simulink model "simdecod5g1"  (R2023b)
settings: Solver=VariableStepAuto  StartTime=0.0  StopTime=0.01  RelTol=1e-3
undefined symbols (not defined in the file): waveform
libraries: commdigbbndam3 x3, commofdm x3
settings Model: Creator=joshua  LastModifiedBy=joshua

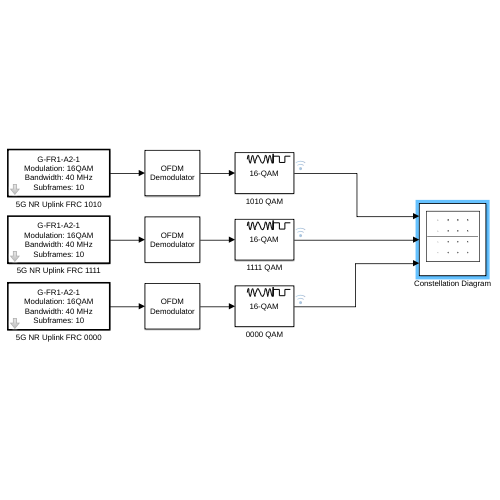
[thumbnail: Simulink's stored preview of the top-level diagram]
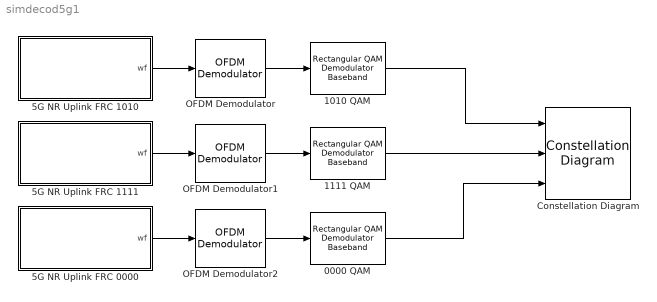
== system simdecod5g1 ==
  "0000 QAM " : commdigbbndam3/Rectangular QAM Demodulator Baseband  M=16  OutType=Bit  DecType=Hard decision  VarSource=Dialog  Variance=1  Dec=Gray  Mapping=[0:15]  PowType=Min. distance between symbols  MinDist=2  AvgPow=1  PeakPow=1  Ph=0  outDtype1=Inherit via internal rule  outDtype2=Inherit via internal rule  derotateFactorWordLen=16  derotateFactorDataTypeStr=Inherit: Same word length as input  derotateFactorLastDataTypeStr=Inherit: Same word length as input  denormFactorWordLen=16  denormFactorDataTypeStr=Inherit: Same word length as input  denormFactorLastDataTypeStr=Inherit: Same word length as input  prodOutWordLen=32  prodOutOverflowMode=Wrap  prodOutRoundingMode=Floor  prodOutOvFlMode=off  prodOutOvFlModeLastStrValue=off  sumWordLen=32
      settings: LibrarySourceBlock=|
      | commhdldigbbndam/Rectangular QAM
      | Demodulator
      | Baseband
  "1010 QAM " : commdigbbndam3/Rectangular QAM Demodulator Baseband  M=16  OutType=Bit  DecType=Hard decision  VarSource=Dialog  Variance=1  Dec=Gray  Mapping=[0:15]  PowType=Min. distance between symbols  MinDist=2  AvgPow=1  PeakPow=1  Ph=0  outDtype1=Inherit via internal rule  outDtype2=Inherit via internal rule  derotateFactorWordLen=16  derotateFactorDataTypeStr=Inherit: Same word length as input  derotateFactorLastDataTypeStr=Inherit: Same word length as input  denormFactorWordLen=16  denormFactorDataTypeStr=Inherit: Same word length as input  denormFactorLastDataTypeStr=Inherit: Same word length as input  prodOutWordLen=32  prodOutOverflowMode=Wrap  prodOutRoundingMode=Floor  prodOutOvFlMode=off  prodOutOvFlModeLastStrValue=off  sumWordLen=32
      settings: LibrarySourceBlock=|
      | commhdldigbbndam/Rectangular QAM
      | Demodulator
      | Baseband
  "1111 QAM " : commdigbbndam3/Rectangular QAM Demodulator Baseband  M=16  OutType=Bit  DecType=Hard decision  VarSource=Dialog  Variance=1  Dec=Gray  Mapping=[0:15]  PowType=Min. distance between symbols  MinDist=2  AvgPow=1  PeakPow=1  Ph=0  outDtype1=Inherit via internal rule  outDtype2=Inherit via internal rule  derotateFactorWordLen=16  derotateFactorDataTypeStr=Inherit: Same word length as input  derotateFactorLastDataTypeStr=Inherit: Same word length as input  denormFactorWordLen=16  denormFactorDataTypeStr=Inherit: Same word length as input  denormFactorLastDataTypeStr=Inherit: Same word length as input  prodOutWordLen=32  prodOutOverflowMode=Wrap  prodOutRoundingMode=Floor  prodOutOvFlMode=off  prodOutOvFlModeLastStrValue=off  sumWordLen=32
      settings: LibrarySourceBlock=|
      | commhdldigbbndam/Rectangular QAM
      | Demodulator
      | Baseband
  5G NR Uplink FRC 0000 : MATLAB Function  Tag=BlockGeneratedWWGApp  TreatAsAtomicUnit=on  SystemSampleTime=1.3020833333333332899e-06  mask(5G NR Uplink FRC Waveform Generator){nsamps=80, OutputAfterFinalValue=Setting to zero}
      mask prompts: nsamps "Samples per frame:"; OutputAfterFinalValue "Form output after final data value by:"
      mask init:
      | %% Generating Uplink FRC waveform
      | % Uplink FRC configuration
      | cfgULFRC = nrULCarrierConfig;
      | cfgULFRC.Label = 'G-FR1-A2-1';
      | cfgULFRC.FrequencyRange = 'FR1';
      | cfgULFRC.ChannelBandwidth = 40;
      | cfgULFRC.NCellID = 1;
      | cfgULFRC.NumSubframes = 10;
      | cfgULFRC.InitialNSubframe = 0;
      | cfgULFRC.WindowingPercent = 0;
      | cfgULFRC.SampleRate = [];
      | cfgULFRC.CarrierFrequency = 0;
      | 
      | %% SCS specific carriers
      | scscarrier = nrSCSCarrierConfig;
      | scscarrier.SubcarrierSpacing = 15;
      | scscarrier.NSizeGrid = 216;
      | scscarrier.NStartGrid = 0;
      | 
      | cfgULFRC.SCSCarriers = {scscarrier};
      | 
      | %% Bandwidth Parts
      | bwp = nrWavegenBWPConfig;
      | bwp.BandwidthPartID = 1;
      | bwp.Label = 'BWP1';
      | bwp.SubcarrierSpacing = 15;
      | bwp.CyclicPrefix = 'normal';
      | bwp.NSizeBWP = 216;
      | bwp.NStartBWP = 0;
      | 
      | cfgULFRC.BandwidthParts = {bwp};
      | 
      | intracellguardbands = nrIntraCellGuardBandsConfig;
      | intracellguardbands.GuardBandSize = zeros(0,2);
      | intracellguardbands.SubcarrierSpacing = 15;
      | 
      | cfgULFRC.IntraCellGuardBands = {intracellguardbands};
      | 
      | %% PUSCH Instances Configuration
      | pusch = nrWavegenPUSCHConfig;
      | pusch.Enable = true;
      | pusch.Label = 'PUSCH sequence for G-FR1-A2-1';
      | pusch.Power = 0;
      | pusch.BandwidthPartID = 1;
      | pusch.Modulation = '16QAM';
      | pusch.NumLayers = 1;
      | pusch.MappingType = 'A';
      | pusch.SymbolAllocation = [0 14];
      | pusch.SlotAllocation = 0:9;
      | pusch.Period = 10;
      | pusch.PRBSet = 95:119;
      | pusch.TransformPrecoding = false;
      | pusch.TransmissionScheme = 'codebook';
      | pusch.NumAntennaPorts = 1;
      | pusch.TPMI = 0;
      | pusch.FrequencyHopping = 'neither';
      | pusch.SecondHopStartPRB = 0;
      | pusch.Interlacing = false;
      | pusch.RBSetIndex = 0;
      | pusch.InterlaceIndex = 0;
      | pusch.NID = [];
      | pusch.RNTI = 1;
      | pusch.NRAPID = [];
      | pusch.Coding = true;
      | pusch.TargetCodeRate = 0.642578125;
      | pusch.XOverhead = 0;
      | pusch.RVSequence = 0;
      | pusch.DataSource = 0*ones([1000 1]);
      | pusch.EnableACK = false;
      | pusch.NumACKBits = 10;
      | pusch.BetaOffsetACK = 20;
      | pusch.DataSourceACK = 'PN9-ITU';
      | pusch.EnableCSI1 = false;
      | pusch.NumCSI1Bits = 10;
      | pusch.BetaOffsetCSI1 = 6.25;
      | pusch.DataSourceCSI1 = 'PN9-ITU';
      | pusch.EnableCSI2 = false;
      | pusch.NumCSI2Bits = 10;
      | pusch.BetaOffsetCSI2 = 6.25;
      | pusch.DataSourceCSI2 = 'PN9-ITU';
      | pusch.EnableCGUCI = false;
      | pusch.NumCGUCIBits = 7;
      | pusch.BetaOffsetCGUCI = 20;
      | pusch.DataSourceCGUCI = 'PN9-ITU';
      | pusch.EnableULSCH = true;
      | pusch.UCIScaling = 1;
      | pusch.DMRSPower = 3;
      | pusch.EnablePTRS = false;
      | pusch.PTRSPower = 0;
      | 
      | % PUSCH DM-RS
      | puschDMRS = nrPUSCHDMRSConfig;
      | puschDMRS.DMRSConfigurationType = 1;
      | puschDMRS.DMRSTypeAPosition = 2;
      | puschDMRS.DMRSAdditionalPosition = 1;
      | puschDMRS.DMRSLength = 1;
      | puschDMRS.CustomSymbolSet = [];
      | puschDMRS.DMRSPortSet = 0;
      | puschDMRS.NIDNSCID = [];
      | puschDMRS.NSCID = 0;
      | puschDMRS.GroupHopping = false;
      | puschDMRS.SequenceHopping = false;
      | puschDMRS.NRSID = [];
      | puschDMRS.NumCDMGroupsWithoutData = 2;
      | puschDMRS.DMRSUplinkR16 = false;
      | puschDMRS.DMRSUplinkTransformPrecodingR16 = false;
      | 
      | pusch.DMRS = puschDMRS;
      | 
      | % PUSCH PT-RS
      | puschPTRS = nrPUSCHPTRSConfig;
      | puschPTRS.TimeDensity = 1;
      | puschPTRS.FrequencyDensity = 2;
      | puschPTRS.NumPTRSSamples = 2;
      | puschPTRS.NumPTRSGroups = 2;
      | puschPTRS.REOffset = '00';
      | puschPTRS.PTRSPortSet = 0;
      | puschPTRS.NID = [];
      | 
      | pusch.PTRS = puschPTRS;
      | 
      | cfgULFRC.PUSCH = {pusch};
      | 
      | %% PUCCH Instances Configuration
      | pucch = nrWavegenPUCCH0Config;
      | pucch.Enable = false;
      | pucch.Label = 'PUCCH format 0';
      | pucch.Power = 0;
      | pucch.BandwidthPartID = 1;
      | pucch.SymbolAllocation = [13 1];
      | pucch.SlotAllocation = 0:9;
      | pucch.Period = 10;
      | pucch.PRBSet = 0;
      | pucch.FrequencyHopping = 'neither';
      | pucch.SecondHopStartPRB = 1;
      | pucch.Interlacing = false;
      | pucch.RBSetIndex = 0;
      | pucch.InterlaceIndex = 0;
      | pucch.GroupHopping = 'neither';
      | pucch.HoppingID = [];
      | pucch.InitialCyclicShift = 0;
      | pucch.NumUCIBits = 1;
      | pucch.DataSourceUCI = 'PN9-ITU';
      | pucch.DataSourceSR = 0;
      | 
      | cfgULFRC.PUCCH = {pucch};
      | 
      | %% SRS Instances Configuration
      | srs = nrWavegenSRSConfig;
      | srs.Enable = false;
      | srs.Label = 'SRS1';
      | srs.Power = 0;
      | srs.BandwidthPartID = 1;
      | srs.NumSRSPorts = 1;
      | srs.SymbolStart = 13;
      | srs.NumSRSSymbols = 1;
      | srs.SlotAllocation = 0:9;
      | srs.Period = 10;
      | srs.FrequencyStart = 0;
      | srs.NRRC = 0;
      | srs.CSRS = 0;
      | srs.BSRS = 0;
      | srs.BHop = 0;
      | srs.Repetition = 1;
      | srs.KTC = 2;
      | srs.KBarTC = 0;
      | srs.FrequencyScalingFactor = 1;
      | srs.StartRBIndex = 0;
      | srs.EnableStartRBHopping = false;
      | srs.CyclicShift = 0;
      | srs.GroupSeqHopping = 'neither';
      | srs.NSRSID = 0;
      | srs.SRSPositioning = false;
      | 
      | cfgULFRC.SRS = {srs};
      | 
      | % Generation
      | [waveform,info] = nrWaveformGenerator(cfgULFRC);
      | 
      | Fs = info.ResourceGrids(1).Info.SampleRate; 								 % Specify the sample rate of the waveform in Hz
      | 
      | %% Configuring block: update parameters and UserData
      | % Get current block
      | thisBlock = gcb;
      | 
      | % Set info parameters
      | maskHandle = Simulink.Mask.get(thisBlock);
      | textFsDialog = maskHandle.getDialogControl('textFs');
      | textFsDialog.Prompt = ['Waveform sample rate (Fs): ' num2str(Fs*1e-6,'%.9g') ' MHz'];
      | textWfLengthDialog = maskHandle.getDialogControl('textWFLength');
      | textWfLengthDialog.Prompt = ['Waveform length: ' num2str(length(waveform)) ' samples'];
      | 
      | % Set sample time of the block
      | set_param(thisBlock, 'SystemSampleTime', num2str(nsamps/Fs,'%.20g'));
      | 
      | % Update UserData
      | outVar.WaveformConfig = cfgULFRC;
      | outVar.WaveformLength = length(waveform);
      | outVar.Fs = Fs;
      | set_param(thisBlock, 'UserData', outVar);
  5G NR Uplink FRC 1010 : MATLAB Function  Tag=BlockGeneratedWWGApp  TreatAsAtomicUnit=on  SystemSampleTime=1.3020833333333332899e-06  mask(5G NR Uplink FRC Waveform Generator){nsamps=80, OutputAfterFinalValue=Setting to zero}
      mask prompts: nsamps "Samples per frame:"; OutputAfterFinalValue "Form output after final data value by:"
      mask init:
      | %% Generating Uplink FRC waveform
      | % Uplink FRC configuration
      | cfgULFRC = nrULCarrierConfig;
      | cfgULFRC.Label = 'G-FR1-A2-1';
      | cfgULFRC.FrequencyRange = 'FR1';
      | cfgULFRC.ChannelBandwidth = 40;
      | cfgULFRC.NCellID = 1;
      | cfgULFRC.NumSubframes = 10;
      | cfgULFRC.InitialNSubframe = 0;
      | cfgULFRC.WindowingPercent = 0;
      | cfgULFRC.SampleRate = [];
      | cfgULFRC.CarrierFrequency = 0;
      | 
      | %% SCS specific carriers
      | scscarrier = nrSCSCarrierConfig;
      | scscarrier.SubcarrierSpacing = 15;
      | scscarrier.NSizeGrid = 216;
      | scscarrier.NStartGrid = 0;
      | 
      | cfgULFRC.SCSCarriers = {scscarrier};
      | 
      | %% Bandwidth Parts
      | bwp = nrWavegenBWPConfig;
      | bwp.BandwidthPartID = 1;
      | bwp.Label = 'BWP1';
      | bwp.SubcarrierSpacing = 15;
      | bwp.CyclicPrefix = 'normal';
      | bwp.NSizeBWP = 216;
      | bwp.NStartBWP = 0;
      | 
      | cfgULFRC.BandwidthParts = {bwp};
      | 
      | intracellguardbands = nrIntraCellGuardBandsConfig;
      | intracellguardbands.GuardBandSize = zeros(0,2);
      | intracellguardbands.SubcarrierSpacing = 15;
      | 
      | cfgULFRC.IntraCellGuardBands = {intracellguardbands};
      | 
      | %% PUSCH Instances Configuration
      | pusch = nrWavegenPUSCHConfig;
      | pusch.Enable = true;
      | pusch.Label = 'PUSCH sequence for G-FR1-A2-1';
      | pusch.Power = 0;
      | pusch.BandwidthPartID = 1;
      | pusch.Modulation = '16QAM';
      | pusch.NumLayers = 1;
      | pusch.MappingType = 'A';
      | pusch.SymbolAllocation = [0 14];
      | pusch.SlotAllocation = 0:9;
      | pusch.Period = 10;
      | pusch.PRBSet = 95:119;
      | pusch.TransformPrecoding = false;
      | pusch.TransmissionScheme = 'codebook';
      | pusch.NumAntennaPorts = 1;
      | pusch.TPMI = 0;
      | pusch.FrequencyHopping = 'neither';
      | pusch.SecondHopStartPRB = 0;
      | pusch.Interlacing = false;
      | pusch.RBSetIndex = 0;
      | pusch.InterlaceIndex = 0;
      | pusch.NID = [];
      | pusch.RNTI = 1;
      | pusch.NRAPID = [];
      | pusch.Coding = true;
      | pusch.TargetCodeRate = 0.642578125;
      | pusch.XOverhead = 0;
      | pusch.RVSequence = 0;
      | pusch.DataSource = [1 0 1 0 1 0 1 0 1 0 1 0 1 0 1 0 1 0 1 0 1 0 1 0 1 0 1 0 1 0 1 0 1 0 1 0 1 0 1 0 1 0 1 0 1 0 1 0 1 0];
      | pusch.EnableACK = false;
      | pusch.NumACKBits = 10;
      | pusch.BetaOffsetACK = 20;
      | pusch.DataSourceACK = 'PN9-ITU';
      | pusch.EnableCSI1 = false;
      | pusch.NumCSI1Bits = 10;
      | pusch.BetaOffsetCSI1 = 6.25;
      | pusch.DataSourceCSI1 = 'PN9-ITU';
      | pusch.EnableCSI2 = false;
      | pusch.NumCSI2Bits = 10;
      | pusch.BetaOffsetCSI2 = 6.25;
      | pusch.DataSourceCSI2 = 'PN9-ITU';
      | pusch.EnableCGUCI = false;
      | pusch.NumCGUCIBits = 7;
      | pusch.BetaOffsetCGUCI = 20;
      | pusch.DataSourceCGUCI = 'PN9-ITU';
      | pusch.EnableULSCH = true;
      | pusch.UCIScaling = 1;
      | pusch.DMRSPower = 3;
      | pusch.EnablePTRS = false;
      | pusch.PTRSPower = 0;
      | 
      | % PUSCH DM-RS
      | puschDMRS = nrPUSCHDMRSConfig;
      | puschDMRS.DMRSConfigurationType = 1;
      | puschDMRS.DMRSTypeAPosition = 2;
      | puschDMRS.DMRSAdditionalPosition = 1;
      | puschDMRS.DMRSLength = 1;
      | puschDMRS.CustomSymbolSet = [];
      | puschDMRS.DMRSPortSet = 0;
      | puschDMRS.NIDNSCID = [];
      | puschDMRS.NSCID = 0;
      | puschDMRS.GroupHopping = false;
      | puschDMRS.SequenceHopping = false;
      | puschDMRS.NRSID = [];
      | puschDMRS.NumCDMGroupsWithoutData = 2;
      | puschDMRS.DMRSUplinkR16 = false;
      | puschDMRS.DMRSUplinkTransformPrecodingR16 = false;
      | 
      | pusch.DMRS = puschDMRS;
      | 
      | % PUSCH PT-RS
      | puschPTRS = nrPUSCHPTRSConfig;
      | puschPTRS.TimeDensity = 1;
      | puschPTRS.FrequencyDensity = 2;
      | puschPTRS.NumPTRSSamples = 2;
      | puschPTRS.NumPTRSGroups = 2;
      | puschPTRS.REOffset = '00';
      | puschPTRS.PTRSPortSet = 0;
      | puschPTRS.NID = [];
      | 
      | pusch.PTRS = puschPTRS;
      | 
      | cfgULFRC.PUSCH = {pusch};
      | 
      | %% PUCCH Instances Configuration
      | pucch = nrWavegenPUCCH0Config;
      | pucch.Enable = false;
      | pucch.Label = 'PUCCH format 0';
      | pucch.Power = 0;
      | pucch.BandwidthPartID = 1;
      | pucch.SymbolAllocation = [13 1];
      | pucch.SlotAllocation = 0:9;
      | pucch.Period = 10;
      | pucch.PRBSet = 0;
      | pucch.FrequencyHopping = 'neither';
      | pucch.SecondHopStartPRB = 1;
      | pucch.Interlacing = false;
      | pucch.RBSetIndex = 0;
      | pucch.InterlaceIndex = 0;
      | pucch.GroupHopping = 'neither';
      | pucch.HoppingID = [];
      | pucch.InitialCyclicShift = 0;
      | pucch.NumUCIBits = 1;
      | pucch.DataSourceUCI = 'PN9-ITU';
      | pucch.DataSourceSR = 0;
      | 
      | cfgULFRC.PUCCH = {pucch};
      | 
      | %% SRS Instances Configuration
      | srs = nrWavegenSRSConfig;
      | srs.Enable = false;
      | srs.Label = 'SRS1';
      | srs.Power = 0;
      | srs.BandwidthPartID = 1;
      | srs.NumSRSPorts = 1;
      | srs.SymbolStart = 13;
      | srs.NumSRSSymbols = 1;
      | srs.SlotAllocation = 0:9;
      | srs.Period = 10;
      | srs.FrequencyStart = 0;
      | srs.NRRC = 0;
      | srs.CSRS = 0;
      | srs.BSRS = 0;
      | srs.BHop = 0;
      | srs.Repetition = 1;
      | srs.KTC = 2;
      | srs.KBarTC = 0;
      | srs.FrequencyScalingFactor = 1;
      | srs.StartRBIndex = 0;
      | srs.EnableStartRBHopping = false;
      | srs.CyclicShift = 0;
      | srs.GroupSeqHopping = 'neither';
      | srs.NSRSID = 0;
      | srs.SRSPositioning = false;
      | 
      | cfgULFRC.SRS = {srs};
      | 
      | % Generation
      | [waveform,info] = nrWaveformGenerator(cfgULFRC);
      | 
      | Fs = info.ResourceGrids(1).Info.SampleRate; 								 % Specify the sample rate of the waveform in Hz
      | 
      | %% Configuring block: update parameters and UserData
      | % Get current block
      | thisBlock = gcb;
      | 
      | % Set info parameters
      | maskHandle = Simulink.Mask.get(thisBlock);
      | textFsDialog = maskHandle.getDialogControl('textFs');
      | textFsDialog.Prompt = ['Waveform sample rate (Fs): ' num2str(Fs*1e-6,'%.9g') ' MHz'];
      | textWfLengthDialog = maskHandle.getDialogControl('textWFLength');
      | textWfLengthDialog.Prompt = ['Waveform length: ' num2str(length(waveform)) ' samples'];
      | 
      | % Set sample time of the block
      | set_param(thisBlock, 'SystemSampleTime', num2str(nsamps/Fs,'%.20g'));
      | 
      | % Update UserData
      | outVar.WaveformConfig = cfgULFRC;
      | outVar.WaveformLength = length(waveform);
      | outVar.Fs = Fs;
      | set_param(thisBlock, 'UserData', outVar);
  5G NR Uplink FRC 1111 : MATLAB Function  Tag=BlockGeneratedWWGApp  TreatAsAtomicUnit=on  SystemSampleTime=1.3020833333333332899e-06  mask(5G NR Uplink FRC Waveform Generator){nsamps=80, OutputAfterFinalValue=Setting to zero}
      mask prompts: nsamps "Samples per frame:"; OutputAfterFinalValue "Form output after final data value by:"
      mask init:
      | %% Generating Uplink FRC waveform
      | % Uplink FRC configuration
      | cfgULFRC = nrULCarrierConfig;
      | cfgULFRC.Label = 'G-FR1-A2-1';
      | cfgULFRC.FrequencyRange = 'FR1';
      | cfgULFRC.ChannelBandwidth = 40;
      | cfgULFRC.NCellID = 1;
      | cfgULFRC.NumSubframes = 10;
      | cfgULFRC.InitialNSubframe = 0;
      | cfgULFRC.WindowingPercent = 0;
      | cfgULFRC.SampleRate = [];
      | cfgULFRC.CarrierFrequency = 0;
      | 
      | %% SCS specific carriers
      | scscarrier = nrSCSCarrierConfig;
      | scscarrier.SubcarrierSpacing = 15;
      | scscarrier.NSizeGrid = 216;
      | scscarrier.NStartGrid = 0;
      | 
      | cfgULFRC.SCSCarriers = {scscarrier};
      | 
      | %% Bandwidth Parts
      | bwp = nrWavegenBWPConfig;
      | bwp.BandwidthPartID = 1;
      | bwp.Label = 'BWP1';
      | bwp.SubcarrierSpacing = 15;
      | bwp.CyclicPrefix = 'normal';
      | bwp.NSizeBWP = 216;
      | bwp.NStartBWP = 0;
      | 
      | cfgULFRC.BandwidthParts = {bwp};
      | 
      | intracellguardbands = nrIntraCellGuardBandsConfig;
      | intracellguardbands.GuardBandSize = zeros(0,2);
      | intracellguardbands.SubcarrierSpacing = 15;
      | 
      | cfgULFRC.IntraCellGuardBands = {intracellguardbands};
      | 
      | %% PUSCH Instances Configuration
      | pusch = nrWavegenPUSCHConfig;
      | pusch.Enable = true;
      | pusch.Label = 'PUSCH sequence for G-FR1-A2-1';
      | pusch.Power = 0;
      | pusch.BandwidthPartID = 1;
      | pusch.Modulation = '16QAM';
      | pusch.NumLayers = 1;
      | pusch.MappingType = 'A';
      | pusch.SymbolAllocation = [0 14];
      | pusch.SlotAllocation = 0:9;
      | pusch.Period = 10;
      | pusch.PRBSet = 95:119;
      | pusch.TransformPrecoding = false;
      | pusch.TransmissionScheme = 'codebook';
      | pusch.NumAntennaPorts = 1;
      | pusch.TPMI = 0;
      | pusch.FrequencyHopping = 'neither';
      | pusch.SecondHopStartPRB = 0;
      | pusch.Interlacing = false;
      | pusch.RBSetIndex = 0;
      | pusch.InterlaceIndex = 0;
      | pusch.NID = [];
      | pusch.RNTI = 1;
      | pusch.NRAPID = [];
      | pusch.Coding = true;
      | pusch.TargetCodeRate = 0.642578125;
      | pusch.XOverhead = 0;
      | pusch.RVSequence = 0;
      | pusch.DataSource = ones([1000 1]);
      | pusch.EnableACK = false;
      | pusch.NumACKBits = 10;
      | pusch.BetaOffsetACK = 20;
      | pusch.DataSourceACK = 'PN9-ITU';
      | pusch.EnableCSI1 = false;
      | pusch.NumCSI1Bits = 10;
      | pusch.BetaOffsetCSI1 = 6.25;
      | pusch.DataSourceCSI1 = 'PN9-ITU';
      | pusch.EnableCSI2 = false;
      | pusch.NumCSI2Bits = 10;
      | pusch.BetaOffsetCSI2 = 6.25;
      | pusch.DataSourceCSI2 = 'PN9-ITU';
      | pusch.EnableCGUCI = false;
      | pusch.NumCGUCIBits = 7;
      | pusch.BetaOffsetCGUCI = 20;
      | pusch.DataSourceCGUCI = 'PN9-ITU';
      | pusch.EnableULSCH = true;
      | pusch.UCIScaling = 1;
      | pusch.DMRSPower = 3;
      | pusch.EnablePTRS = false;
      | pusch.PTRSPower = 0;
      | 
      | % PUSCH DM-RS
      | puschDMRS = nrPUSCHDMRSConfig;
      | puschDMRS.DMRSConfigurationType = 1;
      | puschDMRS.DMRSTypeAPosition = 2;
      | puschDMRS.DMRSAdditionalPosition = 1;
      | puschDMRS.DMRSLength = 1;
      | puschDMRS.CustomSymbolSet = [];
      | puschDMRS.DMRSPortSet = 0;
      | puschDMRS.NIDNSCID = [];
      | puschDMRS.NSCID = 0;
      | puschDMRS.GroupHopping = false;
      | puschDMRS.SequenceHopping = false;
      | puschDMRS.NRSID = [];
      | puschDMRS.NumCDMGroupsWithoutData = 2;
      | puschDMRS.DMRSUplinkR16 = false;
      | puschDMRS.DMRSUplinkTransformPrecodingR16 = false;
      | 
      | pusch.DMRS = puschDMRS;
      | 
      | % PUSCH PT-RS
      | puschPTRS = nrPUSCHPTRSConfig;
      | puschPTRS.TimeDensity = 1;
      | puschPTRS.FrequencyDensity = 2;
      | puschPTRS.NumPTRSSamples = 2;
      | puschPTRS.NumPTRSGroups = 2;
      | puschPTRS.REOffset = '00';
      | puschPTRS.PTRSPortSet = 0;
      | puschPTRS.NID = [];
      | 
      | pusch.PTRS = puschPTRS;
      | 
      | cfgULFRC.PUSCH = {pusch};
      | 
      | %% PUCCH Instances Configuration
      | pucch = nrWavegenPUCCH0Config;
      | pucch.Enable = false;
      | pucch.Label = 'PUCCH format 0';
      | pucch.Power = 0;
      | pucch.BandwidthPartID = 1;
      | pucch.SymbolAllocation = [13 1];
      | pucch.SlotAllocation = 0:9;
      | pucch.Period = 10;
      | pucch.PRBSet = 0;
      | pucch.FrequencyHopping = 'neither';
      | pucch.SecondHopStartPRB = 1;
      | pucch.Interlacing = false;
      | pucch.RBSetIndex = 0;
      | pucch.InterlaceIndex = 0;
      | pucch.GroupHopping = 'neither';
      | pucch.HoppingID = [];
      | pucch.InitialCyclicShift = 0;
      | pucch.NumUCIBits = 1;
      | pucch.DataSourceUCI = 'PN9-ITU';
      | pucch.DataSourceSR = 0;
      | 
      | cfgULFRC.PUCCH = {pucch};
      | 
      | %% SRS Instances Configuration
      | srs = nrWavegenSRSConfig;
      | srs.Enable = false;
      | srs.Label = 'SRS1';
      | srs.Power = 0;
      | srs.BandwidthPartID = 1;
      | srs.NumSRSPorts = 1;
      | srs.SymbolStart = 13;
      | srs.NumSRSSymbols = 1;
      | srs.SlotAllocation = 0:9;
      | srs.Period = 10;
      | srs.FrequencyStart = 0;
      | srs.NRRC = 0;
      | srs.CSRS = 0;
      | srs.BSRS = 0;
      | srs.BHop = 0;
      | srs.Repetition = 1;
      | srs.KTC = 2;
      | srs.KBarTC = 0;
      | srs.FrequencyScalingFactor = 1;
      | srs.StartRBIndex = 0;
      | srs.EnableStartRBHopping = false;
      | srs.CyclicShift = 0;
      | srs.GroupSeqHopping = 'neither';
      | srs.NSRSID = 0;
      | srs.SRSPositioning = false;
      | 
      | cfgULFRC.SRS = {srs};
      | 
      | % Generation
      | [waveform,info] = nrWaveformGenerator(cfgULFRC);
      | 
      | Fs = info.ResourceGrids(1).Info.SampleRate; 								 % Specify the sample rate of the waveform in Hz
      | 
      | %% Configuring block: update parameters and UserData
      | % Get current block
      | thisBlock = gcb;
      | 
      | % Set info parameters
      | maskHandle = Simulink.Mask.get(thisBlock);
      | textFsDialog = maskHandle.getDialogControl('textFs');
      | textFsDialog.Prompt = ['Waveform sample rate (Fs): ' num2str(Fs*1e-6,'%.9g') ' MHz'];
      | textWfLengthDialog = maskHandle.getDialogControl('textWFLength');
      | textWfLengthDialog.Prompt = ['Waveform length: ' num2str(length(waveform)) ' samples'];
      | 
      | % Set sample time of the block
      | set_param(thisBlock, 'SystemSampleTime', num2str(nsamps/Fs,'%.20g'));
      | 
      | % Update UserData
      | outVar.WaveformConfig = cfgULFRC;
      | outVar.WaveformLength = length(waveform);
      | outVar.Fs = Fs;
      | set_param(thisBlock, 'UserData', outVar);
  Constellation Diagram : ConstellationDiagram  NumInputPorts=3  WindowPosition=[358.000000,457.000000,511.000000,468.000000,]  Visible=on  ScopeFrameLocation=window  ReferenceConstellation="{[-0.94868+0.94868i        -0.94868+0.31623i        -0.94868-0.31623i        -0.94868-0.94868i        -0.31623+0.94868i        -0.31623+0.31623i        -0.31623-0.31623i        -0.31623-0.94868i         0.31623+0.94868i         0.31623+0.31623i         0.31623-0.31623i         0.31623-0.94868i         0.94868+0.94868i         0.94868+0.31623i         0.94868-0.31623i         0.94868-0.94868i][-0.94868+0.94868i        -0.94868+0.31623i        -0.94868-0.31623i        -0.94868-0.94868i        -0.31623+0.94868i        -0.31623+0.31623i        -0.31623-0.31623i        -0.31623-0.94868i         0.31623+0.94868i         0.31623+0.31623i         0.31623-0.31623i         0.31623-0.94868i         0.94868+0.94868i         0.94868+0.31623i         0.94868-0.31623i         0.94868-0.94868i][-0.94868+0.94868i        -0.94868+0.31623i        -0.94868-0.31623i        -0.94868-0.94868i        -0.31623+0.94868i        -0.31623+0.31623i        -0.31623-0.31623i        -0.31623-0.94868i         0.31623+0.94868i         0.31623+0.31623i         0.31623-0.31623i         0.31623-0.94868i         0.94868+0.94868i         0.94868+0.31623i         0.94868-0.31623i         0.94868-0.94868i]}"  XLimits=[-1.46,1.46]  YLimits=[-1.38,1.38]  ShowLegend=on
  OFDM Demodulator : commofdm/OFDM Demodulator  StatePerturbationForJacobian=1.0e-05  FFTLength=64  NumGuardBandCarriers=[6; 5]  RemoveDCCarrier=off  PilotOutputPort=off  PilotCarrierIndices=[12; 26; 40; 54]  CyclicPrefixLength=16  OversamplingFactor=1  NumSymbols=1  NumReceiveAntennas=1  SimulateUsing=Interpreted execution
  OFDM Demodulator1 : commofdm/OFDM Demodulator  StatePerturbationForJacobian=1.0e-05  FFTLength=64  NumGuardBandCarriers=[6; 5]  RemoveDCCarrier=off  PilotOutputPort=off  PilotCarrierIndices=[12; 26; 40; 54]  CyclicPrefixLength=16  OversamplingFactor=1  NumSymbols=1  NumReceiveAntennas=1  SimulateUsing=Interpreted execution
  OFDM Demodulator2 : commofdm/OFDM Demodulator  StatePerturbationForJacobian=1.0e-05  FFTLength=64  NumGuardBandCarriers=[6; 5]  RemoveDCCarrier=off  PilotOutputPort=off  PilotCarrierIndices=[12; 26; 40; 54]  CyclicPrefixLength=16  OversamplingFactor=1  NumSymbols=1  NumReceiveAntennas=1  SimulateUsing=Interpreted execution
  wires:
  5G NR Uplink FRC 1010/1(wf) -> OFDM Demodulator/1
  OFDM Demodulator/1 -> "1010 QAM "/1
  5G NR Uplink FRC 0000/1(wf) -> OFDM Demodulator2/1
  5G NR Uplink FRC 1111/1(wf) -> OFDM Demodulator1/1
  OFDM Demodulator1/1 -> "1111 QAM "/1
  OFDM Demodulator2/1 -> "0000 QAM "/1
  "1010 QAM "/1 -> Constellation Diagram/1
  "0000 QAM "/1 -> Constellation Diagram/3
  "1111 QAM "/1 -> Constellation Diagram/2

== matlab function simdecod5g1/5G NR Uplink FRC 1010 ==
  data: wf output; waveform parameter; nsamps parameter; OutputAfterFinalValue parameter
function wf = wfGenerator(waveform, nsamps, OutputAfterFinalValue)

% Create persistent variable
persistent src;

% Preallocate output
wf = complex(zeros(nsamps,size(waveform,2)));

if isempty(src)
    % Get action when signal ends
    if OutputAfterFinalValue == 1
        signalEndAction = 'Cyclic repetition';
    else
        signalEndAction = 'Set to zero';
    end
    
    % Initialize persistent dsp.SignalSource to get current frame
    src = dsp.SignalSource(waveform,nsamps,'SignalEndAction',signalEndAction);
end

% Extract current frame
wf(:,:) = src();

end

== matlab function simdecod5g1/5G NR Uplink FRC 0000 ==
  data: wf output; waveform parameter; nsamps parameter; OutputAfterFinalValue parameter
function wf = wfGenerator(waveform, nsamps, OutputAfterFinalValue)

% Create persistent variable
persistent src;

% Preallocate output
wf = complex(zeros(nsamps,size(waveform,2)));

if isempty(src)
    % Get action when signal ends
    if OutputAfterFinalValue == 1
        signalEndAction = 'Cyclic repetition';
    else
        signalEndAction = 'Set to zero';
    end
    
    % Initialize persistent dsp.SignalSource to get current frame
    src = dsp.SignalSource(waveform,nsamps,'SignalEndAction',signalEndAction);
end

% Extract current frame
wf(:,:) = src();

end

== matlab function simdecod5g1/5G NR Uplink FRC 1111 ==
  data: wf output; waveform parameter; nsamps parameter; OutputAfterFinalValue parameter
function wf = wfGenerator(waveform, nsamps, OutputAfterFinalValue)

% Create persistent variable
persistent src;

% Preallocate output
wf = complex(zeros(nsamps,size(waveform,2)));

if isempty(src)
    % Get action when signal ends
    if OutputAfterFinalValue == 1
        signalEndAction = 'Cyclic repetition';
    else
        signalEndAction = 'Set to zero';
    end
    
    % Initialize persistent dsp.SignalSource to get current frame
    src = dsp.SignalSource(waveform,nsamps,'SignalEndAction',signalEndAction);
end

% Extract current frame
wf(:,:) = src();

end
